simulink model "FOC_ctrl"  (R2025b)
settings: Solver=FixedStepAuto  StartTime=0.0  StopTime=Tstop  FixedStep=p.FastTs  RelTol=1e-3
undefined symbols (not defined in the file): angleDeg, c, Inverter, m, Motor, p, torqueNm, Tstop, we
libraries: simulink x5, fl_lib x4, nesl_utility x3, dspsigops x2, ee_lib x1
(part 2 of 3)

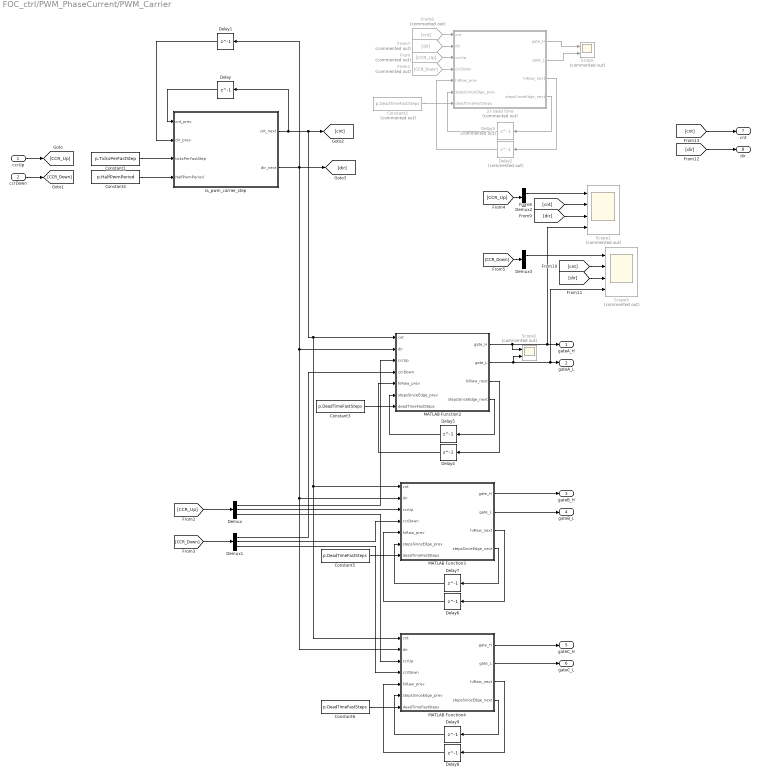
== system FOC_ctrl/PWM_PhaseCurrent/PWM_Carrier ==
  ccrUp : Inport
  ccrDown : Inport  Port=2
  2x dead time : MATLAB Function  Commented=on  TreatAsAtomicUnit=on
  Constant1 : Constant  Value=p.TicksPerFastStep
  Constant2 : Constant  Commented=on  Value=p.DeadTimeFastSteps
  Constant3 : Constant  Value=p.DeadTimeFastSteps
  Constant4 : Constant  Value=p.HalfPwmPeriod
  Constant5 : Constant  Value=p.DeadTimeFastSteps
  Constant6 : Constant  Value=p.DeadTimeFastSteps
  Delay{,4..9} (7 alike) : Delay  DelayLength=1  SampleTime=p.FastTs
  Delay1 : Delay  DelayLength=1  InitialCondition=1  SampleTime=p.FastTs
  Delay2 : Delay  Commented=on  DelayLength=1  SampleTime=p.FastTs
  Delay3 : Delay  Commented=on  DelayLength=1  SampleTime=p.FastTs
  Demux{,1..3} (4 alike) : Demux  Outputs=3
  From : From  Commented=on  GotoTag=CCR_Up
  From1 : From  Commented=on  GotoTag=CCR_Down
  From6 : From  Commented=on  GotoTag=cnt
  From7 : From  Commented=on  GotoTag=dir
  MATLAB Function2 : MATLAB Function  TreatAsAtomicUnit=on
  MATLAB Function3 : MATLAB Function  TreatAsAtomicUnit=on
  MATLAB Function4 : MATLAB Function  TreatAsAtomicUnit=on
  Scope : Scope  Commented=on  NumInputPorts=2
      settings: ActiveDisplayYMinimum=-0.12499999999999997  ActiveDisplayYMaximum=1.125  DataLoggingVariableName=ScopeData14
  Scope1 : Scope  Commented=on  NumInputPorts=4
      settings: ActiveDisplayYMinimum=-9127.6330234277448  ActiveDisplayYMaximum=17916.94761530693  DataLoggingVariableName=ScopeData13
  Scope2 : Scope  Commented=on  NumInputPorts=2
      settings: ActiveDisplayYMinimum=-0.12499999999999997  ActiveDisplayYMaximum=1.125  DataLoggingVariableName=ScopeData21
  Scope5 : Scope  Commented=on  NumInputPorts=4
      settings: ActiveDisplayYMinimum=-665.124999999998  ActiveDisplayYMaximum=5976.1249999999827  DataLoggingVariableName=ScopeData18
  ss_pwm_carrier_step : MATLAB Function  TreatAsAtomicUnit=on
  gateA_H : Outport
  gateA_L : Outport  Port=2
  gateB_H : Outport  Port=3
  gateB_L : Outport  Port=4
  gateC_H : Outport  Port=5
  gateC_L : Outport  Port=6
  cnt : Outport  Port=7
  dir : Outport  Port=8
  wires:
  Constant4/1 -> ss_pwm_carrier_step/4(HalfPwmPeriod)
  Constant1/1 -> ss_pwm_carrier_step/3(ticksPerFastStep)
  Delay/1 -> ss_pwm_carrier_step/1(cnt_prev)
  Delay1/1 -> ss_pwm_carrier_step/2(dir_prev)
  2x dead time/3(hiRaw_next) -> Delay2/1
  Delay2/1 -> 2x dead time/5(hiRaw_prev)
  2x dead time/4(stepsSinceEdge_next) -> Delay3/1
  Delay3/1 -> 2x dead time/6(stepsSinceEdge_prev)
  Constant2/1 -> 2x dead time/7(deadTimeFastSteps)
  2x dead time/1(gate_H) -> Scope/1
  2x dead time/2(gate_L) -> Scope/2
  ccrUp/1 -> [CCR_Up]
  ccrDown/1 -> [CCR_Down]
  From/1 -> 2x dead time/3(ccrUp)
  From1/1 -> 2x dead time/4(ccrDown)
  [CCR_Up] -> Demux/1
  [CCR_Down] -> Demux1/1
  Demux1/1 -> MATLAB Function2/4(ccrDown)
  Demux/1 -> MATLAB Function2/3(ccrUp)
  MATLAB Function2/2(gate_L) -> Scope2/2, Scope5/4, gateA_L/1
  MATLAB Function2/1(gate_H) -> Scope2/1, gateA_H/1, Scope1/4
  Constant3/1 -> MATLAB Function2/7(deadTimeFastSteps)
  Delay5/1 -> MATLAB Function2/6(stepsSinceEdge_prev)
  MATLAB Function2/4(stepsSinceEdge_next) -> Delay5/1
  Delay4/1 -> MATLAB Function2/5(hiRaw_prev)
  MATLAB Function2/3(hiRaw_next) -> Delay4/1
  MATLAB Function3/3(hiRaw_next) -> Delay6/1
  Delay6/1 -> MATLAB Function3/5(hiRaw_prev)
  MATLAB Function3/4(stepsSinceEdge_next) -> Delay7/1
  Delay7/1 -> MATLAB Function3/6(stepsSinceEdge_prev)
  Constant5/1 -> MATLAB Function3/7(deadTimeFastSteps)
  MATLAB Function3/1(gate_H) -> gateB_H/1
  MATLAB Function3/2(gate_L) -> gateB_L/1
  Demux/2 -> MATLAB Function3/3(ccrUp)
  Demux1/2 -> MATLAB Function3/4(ccrDown)
  Demux1/3 -> MATLAB Function4/4(ccrDown)
  Demux/3 -> MATLAB Function4/3(ccrUp)
  MATLAB Function4/2(gate_L) -> gateC_L/1
  MATLAB Function4/1(gate_H) -> gateC_H/1
  Constant6/1 -> MATLAB Function4/7(deadTimeFastSteps)
  Delay9/1 -> MATLAB Function4/6(stepsSinceEdge_prev)
  MATLAB Function4/4(stepsSinceEdge_next) -> Delay9/1
  Delay8/1 -> MATLAB Function4/5(hiRaw_prev)
  MATLAB Function4/3(hiRaw_next) -> Delay8/1
  ss_pwm_carrier_step/2(dir_next) -> [dir], Delay1/1, MATLAB Function2/2(dir), MATLAB Function3/2(dir), MATLAB Function4/2(dir)
  ss_pwm_carrier_step/1(cnt_next) -> MATLAB Function4/1(cnt), MATLAB Function3/1(cnt), MATLAB Function2/1(cnt), [cnt], Delay/1
  [CCR_Up] -> Demux2/1
  [CCR_Down] -> Demux3/1
  Demux2/1 -> Scope1/1
  Demux3/1 -> Scope5/1
  From6/1 -> 2x dead time/1(cnt)
  From7/1 -> 2x dead time/2(dir)
  [cnt] -> Scope1/2
  [dir] -> Scope1/3
  [dir] -> Scope5/3
  [cnt] -> Scope5/2
  [cnt] -> cnt/1
  [dir] -> dir/1

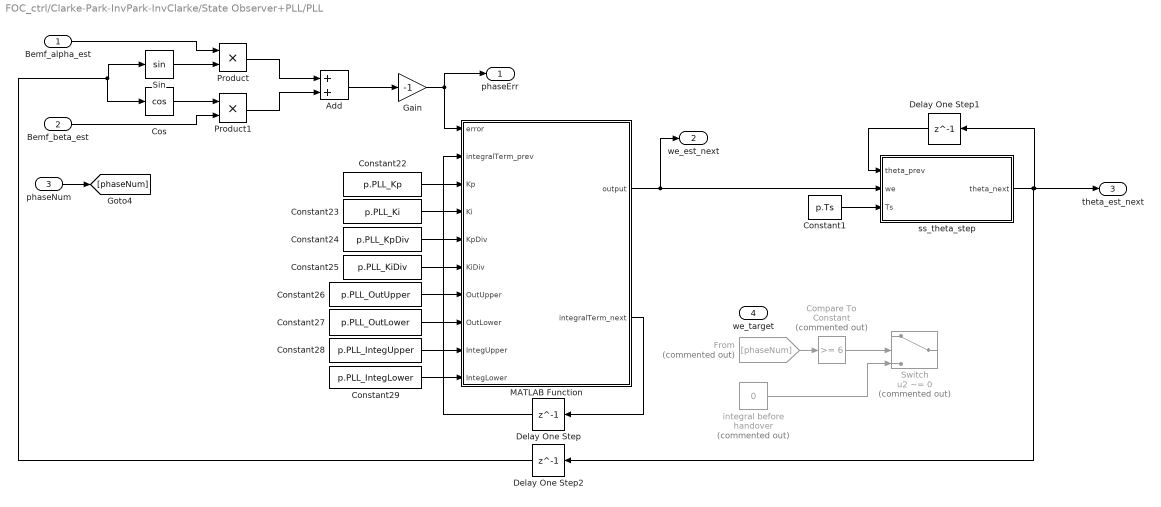
== system FOC_ctrl/Clarke-Park-InvPark-InvClarke/State Observer+PLL/PLL ==
  Bemf_alpha_est : Inport
  Bemf_beta_est : Inport  Port=2
  phaseNum : Inport  Port=3
  we_target : Inport  Port=4
  Add : Sum
  Compare To Constant : simulink/Logic and Bit Operations/Compare To Constant  Commented=on  relop=>=  const=6  OutDataTypeStr=boolean
  Constant1 : Constant  Value=p.Ts
  Constant22 : Constant  Value=p.PLL_Kp
  Constant23 : Constant  Value=p.PLL_Ki
  Constant24 : Constant  Value=p.PLL_KpDiv
  Constant25 : Constant  Value=p.PLL_KiDiv
  Constant26 : Constant  Value=p.PLL_OutUpper
  Constant27 : Constant  Value=p.PLL_OutLower
  Constant28 : Constant  Value=p.PLL_IntegUpper
  Constant29 : Constant  Value=p.PLL_IntegLower
  Cos : Trigonometry  Operator=cos
  Delay One Step : Delay  DelayLength=1
  Delay One Step1 : Delay  DelayLength=1
  Delay One Step2 : Delay  DelayLength=1
  From : From  Commented=on  GotoTag=phaseNum
  Gain : Gain  Gain=-1
  MATLAB Function : MATLAB Function  TreatAsAtomicUnit=on
  Product : Product
  Product1 : Product
  Sin : Trigonometry
  Switch : Switch  Commented=on  Criteria=u2 ~= 0  SaturateOnIntegerOverflow=off  InputSameDT=off
  "integral before handover " : Constant  Commented=on  Value=0
  ss_theta_step : MATLAB Function  TreatAsAtomicUnit=on
  phaseErr : Outport
  we_est_next : Outport  Port=2
  theta_est_next : Outport  Port=3
  wires:
  Add/1 -> Gain/1
  Bemf_beta_est/1 -> Product1/2
  Product1/1 -> Add/2
  Bemf_alpha_est/1 -> Product/1
  Sin/1 -> Product/2
  Product/1 -> Add/1
  Cos/1 -> Product1/1
  Gain/1 -> phaseErr/1, MATLAB Function/1(error)
  Delay One Step2/1 -> Cos/1, Sin/1
  MATLAB Function/2(integralTerm_next) -> Delay One Step/1
  Constant1/1 -> ss_theta_step/3(Ts)
  Delay One Step1/1 -> ss_theta_step/1(theta_prev)
  ss_theta_step/1(theta_next) -> theta_est_next/1, Delay One Step1/1, Delay One Step2/1
  MATLAB Function/1(output) -> we_est_next/1, ss_theta_step/2(we)
  Delay One Step/1 -> MATLAB Function/2(integralTerm_prev)
  Constant29/1 -> MATLAB Function/10(IntegLower)
  Constant28/1 -> MATLAB Function/9(IntegUpper)
  Constant26/1 -> MATLAB Function/7(OutUpper)
  Constant27/1 -> MATLAB Function/8(OutLower)
  Constant25/1 -> MATLAB Function/6(KiDiv)
  Constant24/1 -> MATLAB Function/5(KpDiv)
  Constant23/1 -> MATLAB Function/4(Ki)
  Constant22/1 -> MATLAB Function/3(Kp)
  From/1 -> Compare To Constant/1
  "integral before handover "/1 -> Switch/3
  Compare To Constant/1 -> Switch/2
  phaseNum/1 -> [phaseNum]

== system FOC_ctrl/Cogging Torque/Variant Subsystem/BD Nano ==
  theta : Inport
  BD Nano : MATLAB Function  TreatAsAtomicUnit=on  VariantControl=Option.Product==1
  Gain : Gain  Gain=c.ENABLE_COGGING_TORQUE
  Tcog : Outport
  wires:
  BD Nano/1(Tcog) -> Gain/1
  theta/1 -> BD Nano/1(theta)
  Gain/1 -> Tcog/1

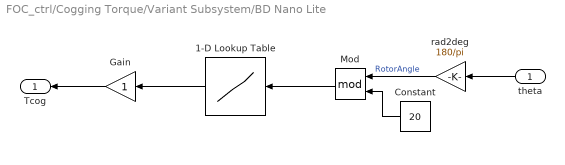
== system FOC_ctrl/Cogging Torque/Variant Subsystem/BD Nano Lite ==
  theta : Inport
  1-D Lookup Table : Lookup_n-D  NumberOfTableDimensions=1  BreakpointsForDimension1=|  BreakpointsForDimension1FirstPoint=0  BreakpointsForDimension1Spacing=0.5  Table=|  InterpMethod=Cubic spline  ExtrapMethod=Cubic spline  InternalRulePriority=Speed  RndMeth=Simplest
      BreakpointsForDimension1=|
      | [0.0
      | 0.5
      | 1.0
      | 1.5
      | 2.0
      | 2.5
      | 3.0
      | 3.5
      | 4.0
      | 4.5
      | 5.0
      | 5.5
      | 6.0
      | 6.5
      | 7.0
      | 7.5
      | 8.0
      | 8.5
      | 9.0
      | 9.5
      | 10.0
      | 10.5
      | 11.0
      | 11.5
      | 12.0
      | 12.5
      | 13.0
      | 13.5
      | 14.0
      | 14.5
      | 15.0
      | 15.5
      | 16.0
      | 16.5
      | 17.0
      | 17.5
      | 18.0
      | 18.5
      | 19.0
      | 19.5
      | 20.0]
      Table=|
      | [0.001
      | 0.002
      | 0.003
      | 0.004
      | 0.005
      | 0.007
      | 0.009
      | 0.011
      | 0.013
      | 0.015
      | 0.017
      | 0.018
      | 0.019
      | 0.018
      | 0.016
      | 0.013
      | 0.010
      | 0.007
      | 0.005
      | 0.003
      | 0.002
      | 0.001
      | 0.000
      | -0.002
      | -0.004
      | -0.007
      | -0.010
      | -0.014
      | -0.017
      | -0.019
      | -0.020
      | -0.019
      | -0.018
      | -0.016
      | -0.014
      | -0.012
      | -0.010
      | -0.008
      | -0.006
      | -0.004
      | -0.001]
  Constant : Constant  Value=20
  Gain : Gain
  Mod : Math  Operator=mod
  rad2deg : Gain  Gain=180/pi
  Tcog : Outport
  wires:
  theta/1 -> rad2deg/1
  1-D Lookup Table/1 -> Gain/1
  Mod/1 -> 1-D Lookup Table/1
  rad2deg/1 -> Mod/1  "RotorAngle"
  Constant/1 -> Mod/2
  Gain/1 -> Tcog/1

== matlab function FOC_ctrl/PWM_PhaseCurrent/get_phase_currents ==
  data: sector input; ia output; iflag input; JDR1 input; JDR2 input; alignFlag input; offset input; convFactorInv input; IaEst input; IbEst input; IcEst input; ib output; ic output
function [ia, ib, ic] = ss_get_phase_currents(sector, iflag, JDR1, JDR2, alignFlag, ...
    offset, convFactorInv, IaEst, IbEst, IcEst)
%SS_GET_PHASE_CURRENTS MATLAB port of R1_GetPhaseCurrents()
% (Src/r1_ps_pwm_curr_fdbk.c, ~lines 463-866).
%
% Reconstructs ia, ib (ic follows from KCL, ia+ib+ic=0) from the two raw
% ADC codes taken this PWM period, using:
%   - sector           : which of the six switching patterns is active
%   - iflag            : IA_OK/IB_OK/IC_OK bits from
%                        ss_calc_duty_and_samplepoints - which of the two
%                        phase currents this sector could sample were
%                        actually inside a wide-enough (>=TMin) window
%   - alignFlag        : true only during the fixed-angle rotor alignment
%                        step at startup (angle pinned to a sector
%                        midpoint, e.g. 30 deg for sector 1) - in that
%                        special case the un-sampled phase's current is
%                        known to be exactly 0 instead of needing an
%                        estimate
%   - IaEst/IbEst/IcEst: fallback current estimates (in the firmware these
%                        come from pwm_curr_fdbk.c's Clarke-transform of
%                        the FOC's own alpha-beta current reference, i.e.
%                        "the current we commanded", used whenever this
%                        period's real sample(s) aren't trustworthy)
%
% Three outcomes per sector, exactly mirroring the C switch/if structure:
%   1) BOTH of the sector's two candidate phases are flagged OK
%        -> both come from real ADC samples this period (best case)
%   2) ONE of the two is flagged OK
%        -> that one is a real sample; the other phase is either forced
%           to 0 (during alignment) or taken from the estimate
%   3) NEITHER is flagged OK
%        -> both phases fall back to the estimate entirely (no real
%           sample was usable this period at all)
%
% JDR1/JDR2 are raw ADC codes (offset not yet removed); convFactorInv is
% CURRENT_CONV_FACTOR_INV (Amps per ADC digit). This port converts to Amps
% immediately after offset removal (wAux1/wAux2), so the branch algebra
% below is unit-for-unit identical to the C source, just already in Amps
% instead of raw int16 digits.

IA_OK = uint8(1); IB_OK = uint8(2); IC_OK = uint8(4);

wAux1 = (double(JDR1) - offset) * convFactorInv;
wAux2 = (double(JDR2) - offset) * convFactorInv;

ia = 0; ib = 0; ic = 0;

switch sector
    case 1
        pair = bitand(iflag, bitor(IA_OK, IC_OK));
        if pair == bitor(IA_OK, IC_OK)
            ia = wAux2; ic = -wAux1; ib = -ia - ic;
        elseif pair ~= 0
            if alignFlag                                   % START Position, 30 deg
                if pair == IA_OK, ia = wAux2; ib = 0; ic = -ia;
                else,             ic = -wAux1; ia = -ic; ib = 0;
                end
            else
                if pair == IA_OK, ia = wAux2; ib = IbEst; ic = -ia - ib;
                else,             ic = -wAux1; ib = IbEst; ia = -ib - ic;
                end
            end
        else
            ia = IaEst; ic = IcEst; ib = -ia - ic;
        end

    case 2
        pair = bitand(iflag, bitor(IB_OK, IC_OK));
        if pair == bitor(IB_OK, IC_OK)
            ib = wAux2; ic = -wAux1; ia = -ib - ic;
        elseif pair ~= 0
            if alignFlag                                   % START Position, 90 deg
                if pair == IB_OK, ib = wAux2; ia = 0; ic = -ib;
                else,             ic = -wAux1; ia = 0; ib = -ic;
                end
            else
                if pair == IB_OK, ib = wAux2; ia = IaEst; ic = -ia - ib;
                else,             ic = -wAux1; ia = IaEst; ib = -ia - ic;
                end
            end
        else
            ib = IbEst; ic = IcEst; ia = -ib - ic;
        end

    case 3
        pair = bitand(iflag, bitor(IA_OK, IB_OK));
        if pair == bitor(IA_OK, IB_OK)
            ib = wAux2; ia = -wAux1;
        elseif pair ~= 0
            if alignFlag                                   % START Position, 150 deg
                if pair == IB_OK, ib = wAux2; ia = -ib;
                else,             ia = -wAux1; ib = -ia;
                end
            else
                if pair == IB_OK, ib = wAux2; ia = IaEst;
                else,             ia = -wAux1; ib = IbEst;
                end
            end
        else
            ib = IbEst; ia = IaEst;
        end
        ic = -ia - ib;  % not computed by the C fn here (ab_t has no `c`); KCL added for convenience

    case 4
        pair = bitand(iflag, bitor(IA_OK, IC_OK));
        if pair == bitor(IA_OK, IC_OK)
            ia = -wAux1; ic = wAux2; ib = -ia - ic;
        elseif pair ~= 0
            if alignFlag                                   % START Position, 210 deg
                if pair == IC_OK, ic = wAux2; ia = -ic; ib = 0;
                else,             ia = -wAux1; ib = 0;
                end
            else
                if pair == IC_OK, ic = wAux2; ib = IbEst; ia = -ib - ic;
                else,             ia = -wAux1; ib = IbEst;
                end
            end
        else
            ic = IcEst; ia = IaEst; ib = -ia - ic;
        end

    case 5
        pair = bitand(iflag, bitor(IB_OK, IC_OK));
        if pair == bitor(IB_OK, IC_OK)
            ib = -wAux1; ic = wAux2; ia = -ib - ic;
        elseif pair ~= 0
            if alignFlag                                   % START Position, 270 deg
                if pair == IC_OK, ic = wAux2; ia = 0; ib = -ic;
                else,             ib = -wAux1; ia = 0;
                end
            else
                if pair == IC_OK, ic = wAux2; ia = IaEst; ib = -ia - ic;
                else,             ib = -wAux1; ia = IaEst;
                end
            end
        else
            ic = IcEst; ib = IbEst; ia = -ib - ic;
        end

    case 6
        pair = bitand(iflag, bitor(IA_OK, IB_OK));
        if pair == bitor(IA_OK, IB_OK)
            ia = wAux2; ib = -wAux1;
        elseif pair ~= 0
            if alignFlag                                   % START Position, 330 deg
                if pair == IA_OK, ia = wAux2; ib = -ia;
                else,             ib = -wAux1; ia = -ib;
                end
            else
                if pair == IA_OK, ia = wAux2; ib = IbEst;
                else,             ib = -wAux1; ia = IaEst;
                end
            end
        else
            ia = IaEst; ib = IbEst;
        end
        ic = -ia - ib;  % not computed by the C fn here (ab_t has no `c`); KCL added for convenience

    otherwise
        error('ss_get_phase_currents:sector', 'sector must be 1..6');
end

end

== matlab function FOC_ctrl/Cogging Torque/Variant Subsystem/BD Nano/BD Nano ==
  data: theta input size=1; Tcog output size=1
function Tcog = fcn(theta)

Tcog = 0.039*sin(18*theta);

== matlab function FOC_ctrl/PWM_PhaseCurrent/ADC_trigger ==
  data: cnt input; trig1 output; dir input; SamplePoint1 input; SamplePoint2 input; ticksPerFastStep input; trig2 output
function [trig1, trig2] = ss_adc_trigger_step(cnt, dir, SamplePoint1, SamplePoint2, ticksPerFastStep)
%SS_ADC_TRIGGER_STEP One fast-rate (p.FastTs) step of the TIM1 CH5/CH6 ->
% TRGO2 -> ADC-injected-trigger chain. Replaces the "SamplePoint changed"
% detector, which fired both triggers simultaneously at the period boundary.
%
% ---------------------------------------------------------------------------
% What the hardware actually does (verified against this build's firmware)
% ---------------------------------------------------------------------------
% Src/main.c, MX_TIM1_Init():
%   CounterMode        = TIM_COUNTERMODE_CENTERALIGNED2
%   CH5, CH6 OCMode    = TIM_OCMODE_PWM2      <-- note: PWM mode *2*
%   MasterOutputTrigger2 = TIM_TRGO2_OC5REF_RISING_OC6REF_RISING
% Src/main.c, ADC2 injected config:
%   ExternalTrigInjecConv = ADC_EXTERNALTRIGINJEC_T1_TRGO, 2 conversions
% Src/r1_ps_pwm_curr_fdbk.c, R1_CalcDutyCycles() (~line 1259):
%   CCR5 = SamplePoint1,  CCR6 = SamplePoint2
%
% In PWM mode 2 the reference OCxREF is LOW while CNT < CCRx and HIGH while
% CNT > CCRx. So an OCxREF *rising* edge is an UP-COUNT crossing of CCRx.
% Both conversions therefore happen in the UP-COUNTING half of the
% center-aligned period, SamplePoint1 first (it is the lower value), then
% SamplePoint2 -> injected rank 1 = JDR1 = SamplePoint1, rank 2 = JDR2 =
% SamplePoint2. That is exactly the pairing ss_get_phase_currents assumes
% (JDR1 -> low-duty phase, JDR2 -> high-duty phase).
%
% This also explains the asymmetric shift: aShiftval is applied +shift in the
% up half (DmaBuffCCR[0:2]) and -shift in the down half (DmaBuffCCR[4:6]), and
% is only ever applied to the max- or min-duty phase, never the mid one. The up
% half is where the shift WIDENS both sampling windows; the down half pays it
% back so the average duty (= commanded voltage) is unchanged. Nothing is
% sampled in the down half, so the narrowed windows there do not matter.
%
% ---------------------------------------------------------------------------
% Why the sample point must be snapped DOWN to the fast grid
% ---------------------------------------------------------------------------
% The simulated carrier only takes values that are multiples of
% ticksPerFastStep (= p.TicksPerFastStep, 170 ticks = 1 us at the current
% settings), so the gate edges - and therefore the real sampling windows in
% the simulation - are quantized to that grid too.
%
% SamplePoint1 = CCR_mid - TSample sits only TSample = 41 ticks (0.24 fast
% steps) below the mid-phase edge. If you fire on the FIRST grid point at or
% after SamplePoint1, that grid point coincides with the mid-phase edge
% whenever (CCR_mid mod ticksPerFastStep) > TSample - i.e. 76% of the time -
% and you sample the wrong window, inside the dead time.
%
% Firing on the LAST grid point at or before the sample point instead is
% provably inside the correct window for every duty pattern the firmware
% flags as valid (windows are guaranteed >= TMin = 415 ticks wide, and
% snapping down costs at most ticksPerFastStep-1 = 169 ticks). Run
% ss_adc_timing_report to re-verify this after any change to PWM_FREQUENCY,
% p.PwmCarrierSamplesPerPeriod or p.DeadTime_ns.
%
% ---------------------------------------------------------------------------
% Inputs / outputs
% ---------------------------------------------------------------------------
% cnt, dir          : ss_pwm_carrier_step.m outputs, THIS fast step
% SamplePoint1/2    : ss_calc_duty_and_samplepoints.m outputs, in timer ticks,
%                     held constant over the PWM period (p.Ts rate signal,
%                     zero-order-held into this fast-rate subsystem)
% ticksPerFastStep  : p.TicksPerFastStep
%
% trig1, trig2      : one-fast-step pulses for the two Sample and Hold
%                     blocks (JDR1 <- trig1, JDR2 <- trig2). No state is
%                     needed: each sample point is bracketed by exactly one
%                     up-count step, so each pulse fires exactly once per
%                     PWM period.
%
% NOTE: the gate vector reaches the Simscape inverter one fast step late
% (Delay6elements at the model root), so Vamp_out at step k reflects the
% carrier value at step k-1. Delay trig1/trig2 by p.AdcTrigAlignSteps fast
% steps OUTSIDE this function to line them up - see the header of
% ss_adc_timing_report for how to check the alignment on a scope.

upCounting = dir > 0;

trig1 = upCounting && (cnt <= SamplePoint1) && ((cnt + ticksPerFastStep) > SamplePoint1);
trig2 = upCounting && (cnt <= SamplePoint2) && ((cnt + ticksPerFastStep) > SamplePoint2);

end

== matlab function FOC_ctrl/Clarke-Park-InvPark-InvClarke/Park ==
  data: Ialpha input; Id output; Ibeta input; theta input; Iq output
function [Id, Iq] = ss_park(Ialpha, Ibeta, theta)
%SS_PARK MATLAB port of MCM_Park() (Src/mc_math.c, ~lines 143-239).
%
% Same sin/cos role-swap as the firmware (Iq uses cos, Id uses sin) -
% verified as the exact inverse of ss_rev_park.m under this convention
% (see ss_clarke.m header). theta is the rotor electrical angle in
% radians (the firmware's Theta is the same angle in Q1.15 format via a
% trig LUT - using cos/sin directly here is the floating-point
% equivalent).
%
% Ialpha, Ibeta : stationary frame currents (ss_clarke.m output)
% theta         : rotor electrical angle, radians
% Id, Iq        : synchronous (rotor) frame currents

c = cos(theta);
s = sin(theta);

Iq = Ialpha * c - Ibeta * s;
Id = Ialpha * s + Ibeta * c;

end

== matlab function FOC_ctrl/Clarke-Park-InvPark-InvClarke/Clarke ==
  data: Ia input; Ialpha output; Ib input; Ibeta output
function [Ialpha, Ibeta] = ss_clarke(Ia, Ib)
%SS_CLARKE MATLAB port of MCM_Clarke() (Src/mc_math.c, ~lines 71-100).
%
% Note this firmware's beta axis is flipped in sign relative to the
% "textbook" amplitude-invariant Clarke transform (which would be
% Ibeta = +(Ia+2*Ib)/sqrt(3)) - this is a deliberate, consistent ST
% convention: MCM_Park/MCM_Rev_Park are written to be exact inverses of
% each other under THIS sign (verified algebraically), so as long as
% ss_park.m / ss_rev_park.m match it too, the closed loop is self-
% consistent - only the direction label ("beta") differs from other
% textbooks, not the actual closed-loop behavior.
%
% Ia, Ib : measured phase currents (from the single-shunt reconstruction,
%          i.e. this model's Ia/Ib outputs)
% Ialpha, Ibeta : stationary (alpha-beta) frame currents

Ialpha = Ia;
Ibeta  = -(Ia + 2*Ib) / sqrt(3);

end

== matlab function FOC_ctrl/Clarke-Park-InvPark-InvClarke/rev_park ==
  data: Vd input; Valpha output; Vq input; theta input; Vbeta output
function [Valpha, Vbeta] = ss_rev_park(Vd, Vq, theta)
%SS_REV_PARK MATLAB port of MCM_Rev_Park() (Src/mc_math.c, ~lines
% 258-297): Valpha = Vq*cos(theta) + Vd*sin(theta)
%           Vbeta  = -Vq*sin(theta) + Vd*cos(theta)
%
% Exact inverse of ss_park.m under the same convention (verified when
% Park was written: Rev_Park(Park(Ialpha,Ibeta,theta),theta) = Ialpha,
% Ibeta for any theta).
%
% Vd, Vq : synchronous-frame voltage commands (PI controller outputs,
%          already converted to per-unit via p.VoltageFullScale)
% theta  : rotor electrical angle, radians (same theta fed to ss_park.m)

c = cos(theta);
s = sin(theta);

Valpha = Vq * c + Vd * s;
Vbeta  = -Vq * s + Vd * c;

end

== matlab function FOC_ctrl/Clarke-Park-InvPark-InvClarke/inv_clarke(V) ==
  data: Valpha input; Va output; Vbeta input; Vb output; Vc output
function [Va, Vb, Vc] = ss_inv_clarke(Valpha, Vbeta)
%SS_INV_CLARKE Inverse Clarke transform - NOT a firmware port (the real
% MCSDK has no such function: PWMC_SetPhaseVoltage() computes SVM duty
% directly from alpha-beta via the fixed-point wX/wY/wZ method, never
% forming Va/Vb/Vc explicitly). This is the bridge WE need because
% ss_svpwm_minmax.m (the SVPWM stage already validated in this build)
% works in the three-phase domain rather than being a byte-for-byte port
% of that alpha-beta-native method (see ss_sector_from_duty.m header).
%
% Derived as the exact algebraic inverse of ss_clarke.m's specific sign
% convention (Ibeta = -(Ia+2*Ib)/sqrt(3), i.e. flipped vs. the "textbook"
% Clarke transform) - NOT copied from a generic inverse-Clarke formula,
% to guarantee round-tripping through ss_clarke.m -> ss_park.m ->
% ss_rev_park.m -> here reproduces the original three phases exactly.
% Verified: ss_inv_clarke(ss_clarke(Ia,Ib)) == [Ia, Ib, Ic] for any Ia,Ib.
%
% Valpha, Vbeta : ss_rev_park.m output (per-unit stationary-frame voltage)
% Va, Vb, Vc    : per-unit three-phase reference voltage, same scale/sign
%                 convention as the Va/Vb/Vc already feeding
%                 ss_svpwm_minmax.m

Va = Valpha;
Vb = -Valpha/2 - (sqrt(3)/2) * Vbeta;
Vc = -Valpha/2 + (sqrt(3)/2) * Vbeta;

end

== matlab function FOC_ctrl/Clarke-Park-InvPark-InvClarke/Startup/the phase sequencer_Updated ==
  data: t_elapsed input; we_target output; Idref_phase output; Iqref_phase output; phaseNum output; p parameter
function [we_target, Idref_phase, Iqref_phase, phaseNum] = ss_startup_sequencer(t_elapsed, p)
%SS_STARTUP_SEQUENCER Smooth-transition startup sequencer for loaded motor
%
% Phase Breakdown:
%   Phase 1 (Align)       : 0.000 - 0.200 s | Holds 0 RPM | Id = 10A, Iq = 0A
%   Phase 1.5 (Transition): 0.200 - 0.220 s | Holds 0 RPM | Id ramps 10A->0A, Iq ramps 0A->10A
%   Phase 2 (Ramp/Acc)    : 0.220 - 0.620 s | Ramps to 2500 RPM | Iq tapers 10A->8A
%   Phase 3               : 0.620 - 0.621 s | Ramps to 2510 RPM | Iq = 8A
%   Phase 4               : 0.621 - 0.622 s | Ramps to 2520 RPM | Iq = 8A
%   Phase 5               : 0.622 - 0.623 s | Ramps to 2530 RPM | Iq = 8A
%   Phase 6               : > 0.623 s       | Ready for closed-loop handover

rpm2we = (2*pi/60) * p.MotorPolePairs;
we_bkpts = p.Startup_RPM * rpm2we;
t_bkpts  = [0, p.Startup_T];

% 1. Command open-loop target electrical speed (we_target)
t_clamped = min(t_elapsed, p.Startup_T(end));
we_target = interp1(t_bkpts, we_bkpts, t_clamped, 'linear');

% 2. Current Reference and Phase State Machine
T_align = p.Startup_T(1); % End of pure align
T_blend = p.Startup_T(2); % End of Id -> Iq blend duration

if t_elapsed <= T_align
    % --- PHASE 1: Pure Alignment (DC Lock) ---
    phaseNum = 1;
    Idref_phase = p.Startup_Id_A;
    Iqref_phase = 0;

elseif t_elapsed <= T_blend
    % --- PHASE 1.5: Smooth Vector Blend (Soft-Transfer at Standstill) ---
    phaseNum = 1.5;
    % Normalized alpha factor going from 0 -> 1 over the blend time
    alpha = (t_elapsed - T_align) / (T_blend - T_align);
    
    % Smooth cross-fade between Id and Iq to avoid current step spikes
    Idref_phase = (1 - alpha) * p.Startup_Id_A;
    Iqref_phase = alpha * p.Startup_Iq_Breakaway_A;

elseif t_elapsed <= p.Startup_T(3)
    % --- PHASE 2: Main Acceleration Ramp ---
    phaseNum = 2;
    Idref_phase = 0;
    
    % Taper Iq down from Breakaway Torque (10A) to Running Startup Torque (4A)
    % as speed increases and static friction drops to dynamic friction
    T_ramp_start = T_blend;
    T_ramp_end   = p.Startup_T(3);
    beta = (t_elapsed - T_ramp_start) / (T_ramp_end - T_ramp_start);
    
    Iqref_phase = (1 - beta) * p.Startup_Iq_Breakaway_A + beta * p.Startup_Iq_A;

elseif t_elapsed <= p.Startup_T(4)
    % --- PHASE 3 ---
    phaseNum = 3;
    Idref_phase = 0;
    Iqref_phase = p.Startup_Iq_A;

elseif t_elapsed <= p.Startup_T(5)
    % --- PHASE 4 ---
    phaseNum = 4;
    Idref_phase = 0;
    Iqref_phase = p.Startup_Iq_A;

elseif t_elapsed <= p.Startup_T(6)
    % --- PHASE 5 ---
    phaseNum = 5;
    Idref_phase = 0;
    Iqref_phase = p.Startup_Iq_A;

else
    % --- PHASE 6: Observer Handoff Ready ---
    phaseNum = 6;
    Idref_phase = 0;
    Iqref_phase = p.Startup_Iq_A; % Holds constant; superseded by Speed Loop Iqref once closed
end

end

== matlab function FOC_ctrl/Clarke-Park-InvPark-InvClarke/State Observer+PLL/MATLAB Function ==
  data: we_est input; speedErrPct output; we_target input; tolFrac input; isConverged output
function [speedErrPct, isConverged] = check_convergence(we_est, we_target, tolFrac)
% tolFrac: e.g. 0.05 for 5%
if abs(we_target) > 50   % avoid a meaningless % error near standstill
    speedErrPct = abs(we_est - we_target) / abs(we_target) * 100;
else
    speedErrPct = 999;    % force "not converged" at/near standstill
end
isConverged = speedErrPct < (tolFrac*100);
end

== matlab function FOC_ctrl/Clarke-Park-InvPark-InvClarke/CalcPhaseCurrentsEst ==
  data: Iq input; IaEst output; Id input; IqAvg_prev input; IdAvg_prev input; theta input; IbEst output; IcEst output; IqAvg_next output; IdAvg_next output; p parameter
function [IaEst, IbEst, IcEst, IqAvg_next, IdAvg_next] = ...
    ss_calc_phase_currents_est(Iq, Id, IqAvg_prev, IdAvg_prev, theta, p)
%SS_CALC_PHASE_CURRENTS_EST MATLAB port of PWMC_CalcPhaseCurrentsEst()
% (Src/pwm_curr_fdbk.c, ~lines 489-529), called once per PWM period from
% Src/mc_tasks_foc.c:787 - the real firmware's replacement for a naive
% sample-and-hold fallback estimate.
%
% NOT built from the current reference (a simplification I mistakenly
% described earlier) - it's built from the MEASURED Iq/Id (this period's
% ss_park output, i.e. the just-reconstructed current), lightly low-pass
% filtered, then rotated back through Rev_Park + inverse-Clarke into an
% a/b/c estimate. This gives a smoother, more physically continuous
% fallback than repeating a single stale sample, without needing to know
% anything about what the controller commanded.
%
% PWMC_LowPassFilter()'s Q15 fixed-point accumulator recursion simplifies
% (once you divide through by the 32768 scaling) to the standard
% exponential filter used here: Y[k] = Y[k-1] + alpha*(in[k]-Y[k-1]),
% alpha = p.LPFAlpha (~0.5 - LPF_FILT_CONST/32768 - a light filter, not
% heavy smoothing).
%
% ss_rev_park.m and ss_inv_clarke.m are reused as-is: Rev_Park is just a
% rotation (works on filtered Id/Iq exactly like it works on PI voltage
% output), and the firmware's temp1/temp2 "Reverse Clarke" formula here
% is, term for term, identical to ss_inv_clarke.m (already verified when
% that file was written).
%
% TIMING: in the C code, PWMC_GetPhaseCurrents() (which reads
% pHandle->IaEst) runs BEFORE PWMC_CalcPhaseCurrentsEst() (which writes
% it) within the same period - so GetPhaseCurrents always sees LAST
% period's estimate, never this period's freshly computed one. Replicate
% this by feeding IaEst/IbEst/IcEst back into ss_get_phase_currents.m
% through a Unit Delay (Z^-1), NOT directly - otherwise this creates the
% same zero-delay algebraic loop we already had to fix once for the
% Vd/Vq path.
%
% Iq, Id             : measured synchronous-frame current (ss_park output,
%                      THIS period)
% IqAvg_prev/IdAvg_prev : filter state - feed back through two Unit Delay
%                      (Z^-1) blocks, initial condition 0
% theta              : rotor electrical angle, radians (same theta used
%                      elsewhere - the real firmware uses hElAngle with an
%                      extra speed-compensation term here that this
%                      simplified open-loop-theta build doesn't model)
%
% IaEst,IbEst,IcEst  : feed through THREE MORE Unit Delay (Z^-1) blocks
%                      before wiring into ss_get_phase_currents.m's
%                      IaEst/IbEst/IcEst inputs (see TIMING note above)
% IqAvg_next/IdAvg_next : feed back to IqAvg_prev/IdAvg_prev next period

IqAvg_next = IqAvg_prev + p.LPFAlpha * (Iq - IqAvg_prev);
IdAvg_next = IdAvg_prev + p.LPFAlpha * (Id - IdAvg_prev);

[Ialpha_est, Ibeta_est] = ss_rev_park(IdAvg_next, IqAvg_next, theta);
[IaEst, IbEst, IcEst] = ss_inv_clarke(Ialpha_est, Ibeta_est);

end

== matlab function FOC_ctrl/Clarke-Park-InvPark-InvClarke/State Observer+PLL/PLL/MATLAB Function ==
  data: error input; integralTerm_prev input; Kp input; Ki input; KpDiv input; KiDiv input; OutUpper input; OutLower input; IntegUpper input; IntegLower input; output output; integralTerm_next output
function [output, integralTerm_next] = ss_pi_controller(error, integralTerm_prev, ...
    Kp, Ki, KpDiv, KiDiv, OutUpper, OutLower, IntegUpper, IntegLower)
%SS_PI_CONTROLLER MATLAB port of PI_Controller()
% (MCSDK_v6.4.2-Full/MotorControl/MCSDK/MCLib/Any/Src/pid_regulator.c,
% ~lines 622-738). Used for both the Id and Iq current loops (same
% function, different gains - matches how the firmware reuses one
% PI_Controller() for pPIDId[M1] and pPIDIq[M1]).
%
% Structure: proportional term, integral term (accumulated then clamped
% to [IntegLower,IntegUpper] BEFORE being added to the proportional
% term), summed and clamped to [OutLower,OutUpper] - then, distinctively,
% whatever amount was clamped off ("discharge") is fed back and added to
% the stored integral term. That's back-calculation anti-windup: it stops
% the integrator winding up further while the output is saturated,
% without needing a separate windup-detection flag.
%
% NOT ported: the C code's wIntegral_sum_temp int32-overflow guards
% (lines ~654-689) - those exist to protect a 32-bit fixed-point
% accumulator from wrapping around, which isn't a concern in double-
% precision floating point. The control algorithm itself (this function)
% is unaffected by omitting them.
%
% integralTerm_prev/integralTerm_next : the PI's stored integral state
% (pHandle->wIntegralTerm) - feed back through a Unit Delay (Z^-1),
% initial condition 0, same pattern as IaEst/IbEst/IcEst and theta_prev
% elsewhere in this build.
%
% error : reference - measured, in the SAME units the gains were tuned
%         for - i.e. raw ADC-digit-equivalent current, NOT Amps (see
%         ss_params.m's "Current-loop PI gains" section for the Amps<->
%         digit and per-unit-voltage<->raw conversions to do at the call
%         site).
% Kp, Ki, KpDiv, KiDiv, OutUpper, OutLower, IntegUpper, IntegLower :
%         p.IQ_* / p.ID_* / p.PI_* from ss_params.m

propTerm = Kp * error;

if Ki == 0
    integralTerm = 0;
else
    integralSum = integralTerm_prev + Ki * error;
    if integralSum > IntegUpper
        integralTerm = IntegUpper;
    elseif integralSum < IntegLower
        integralTerm = IntegLower;
    else
        integralTerm = integralSum;
    end
end

output_raw = propTerm / KpDiv + integralTerm / KiDiv;

discharge = 0;
if output_raw > OutUpper
    discharge = OutUpper - output_raw;
    output = OutUpper;
elseif output_raw < OutLower
    discharge = OutLower - output_raw;
    output = OutLower;
else
    output = output_raw;
end

integralTerm_next = integralTerm + discharge * KiDiv;

end

== matlab function FOC_ctrl/Clarke-Park-InvPark-InvClarke/Startup/handover_timing_gate ==
  data: we_est input; T5_eff output; we_target input; t_elapsed input; tolFrac input; minRampTime input; timeoutMargin input; T5_fixed input; minSpeed input; Count output
function [T5_eff, Count]= handover_timing_gate(we_est, we_target, t_elapsed, tolFrac, minRampTime, timeoutMargin, T5_fixed, minSpeed)
persistent okCount tLatched
if isempty(okCount)
    okCount  = 0;
    tLatched = -1;
end

DEBOUNCE_N = 20;  % consecutive in-tolerance samples required (~1.6ms @ 12.5kHz)

if t_elapsed >= minRampTime && abs(we_target) > 50 && abs(we_est) > minSpeed
    speedErrPct = abs(we_est - we_target) / abs(we_target) * 100;
    if speedErrPct < tolFrac*100
        okCount = okCount + 1;
    else
        okCount = 0;
    end
else
    okCount = 0;
end
Count=okCount;
if tLatched < 0 && okCount >= DEBOUNCE_N
    tLatched = t_elapsed;          % latch the instant convergence was confirmed
end

if tLatched < 0 && okCount >= DEBOUNCE_N
    tLatched = t_elapsed;                   % genuine convergence, latched
elseif tLatched < 0 && t_elapsed >= (T5_fixed + timeoutMargin)
    tLatched = T5_fixed + timeoutMargin;    % timeout fallback, latched to a FIXED point
end

if tLatched >= 0
    T5_eff = tLatched;
else
    T5_eff = 1e6;
end

end

== matlab function FOC_ctrl/Clarke-Park-InvPark-InvClarke/modulation_index(Investigation only) ==
  data: Va input; m output; Vb input; Vc input
function m = ss_modulation_index(Va, Vb, Vc)
%SS_MODULATION_INDEX Voltage vector magnitude (the effective modulation
% index "m") recovered from the three per-unit phase voltages feeding
% ss_svpwm_minmax.m - a diagnostic, not a firmware port.
%
% Derived as the algebraic inverse of ss_inv_clarke.m's specific
% convention (Va=Valpha, Vb=-Valpha/2-sqrt(3)/2*Vbeta,
% Vc=-Valpha/2+sqrt(3)/2*Vbeta => Vbeta=(Vc-Vb)/sqrt(3)), NOT a generic
% formula, so it stays consistent with this build's sign convention.
%
% Simpler equivalent (no need to wait until after InvClarke): since
% ss_rev_park.m is a pure rotation, it preserves vector magnitude, so
% m = sqrt(Vd^2+Vq^2) computed directly from the (per-unit) PI outputs
% gives the exact same number - check there instead if it's more
% convenient to scope.
%
% Guide values: m <= 1.0 is the plain sine-triangle linear range;
% 1.0 < m <= 2/sqrt(3) ~= 1.1547 is the extended range the min-max
% injection in ss_svpwm_minmax.m buys you (six-step limit); m above that
% means the commanded voltage vector can no longer be tracked - the
% actual output will be less than/distorted relative to what was
% commanded (overmodulation).

Valpha = Va;
Vbeta = (Vc - Vb) / sqrt(3);

m = sqrt(Valpha.^2 + Vbeta.^2);

end

== matlab function FOC_ctrl/PWM_PhaseCurrent/PWM_Carrier/ss_pwm_carrier_step ==
  data: cnt_prev input; cnt_next output; dir_prev input; ticksPerFastStep input; HalfPwmPeriod input; dir_next output
function [cnt_next, dir_next] = ss_pwm_carrier_step(cnt_prev, dir_prev, ticksPerFastStep, HalfPwmPeriod)
%SS_PWM_CARRIER_STEP One fast-rate (p.FastTs) step of the real TIM1
% center-aligned up-down counter, running underneath the whole p.Ts-rate
% model - NOT a firmware port (the real counter is free-running hardware,
% not software), just this simulation's stand-in for it.
%
% Advances the counter by ticksPerFastStep each fast step and reflects
% direction at 0 and HalfPwmPeriod, producing the same triangle-wave
% counter TIM1 actually runs (0 -> HalfPwmPeriod -> 0, repeating every
% p.Ts). Run this in a subsystem at p.FastTs (see ss_params.m's "PWM
% carrier" section) - NOT at the model's main p.Ts rate.
%
% cnt_prev, dir_prev : counter state (ticks, +1/-1) - feed back through
%                       two Unit Delay (Z^-1) blocks AT THE FAST RATE,
%                       initial condition cnt=0, dir=+1
% ticksPerFastStep    : p.TicksPerFastStep
% HalfPwmPeriod       : p.HalfPwmPeriod (ARR, timer ticks)

cnt_raw = cnt_prev + dir_prev * ticksPerFastStep;

if cnt_raw >= HalfPwmPeriod
    cnt_next = HalfPwmPeriod - (cnt_raw - HalfPwmPeriod);
    dir_next = -1;
elseif cnt_raw <= 0
    cnt_next = -cnt_raw;
    dir_next = 1;
else
    cnt_next = cnt_raw;
    dir_next = dir_prev;
end

end

== matlab function FOC_ctrl/PWM_PhaseCurrent/PWM_Carrier/2x dead time ==
  data: cnt input; gate_H output; dir input; ccrUp input; ccrDown input; hiRaw_prev input double; stepsSinceEdge_prev input double; deadTimeFastSteps input; gate_L output; hiRaw_next output; stepsSinceEdge_next output
function [gate_H, gate_L, hiRaw_next, stepsSinceEdge_next] = ss_pwm_gate_step( ...
    cnt, dir, ccrUp, ccrDown, hiRaw_prev, stepsSinceEdge_prev, deadTimeFastSteps)
%SS_PWM_GATE_STEP One fast-rate (p.FastTs) step of a single phase's
% high/low-side switch state, matching STM32 timer PWM mode 1 (active
% while counter < compare value, regardless of counting direction) with
% dead-time inserted around every transition.
%
% Call this once per phase (A/B/C) each fast step - each phase has its
% own hiRaw_prev/stepsSinceEdge_prev state, fed back through Unit Delay
% (Z^-1) blocks AT THE FAST RATE, initial condition hiRaw=false,
% stepsSinceEdge=deadTimeFastSteps (so the very first step isn't wrongly
% held in a dead zone).
%
% This is a genuinely stateful, one-fast-step-at-a-time replacement for
% ss_pwm_waveform.m's batch/offline NxN dead-time trick - simpler and
% more natural now that this runs as part of the live simulation instead
% of a one-shot reconstruction: "how many fast steps since the last
% transition" is just a counter, no need to find edges after the fact.
%
% cnt, dir            : ss_pwm_carrier_step.m output, this fast step
% ccrUp, ccrDown       : this phase's compare value for the up-count/
%                        down-count half (ss_calc_duty_and_samplepoints.m's
%                        DmaBuffCCR_up(k)/DmaBuffCCR_down(k), HELD constant
%                        across the whole PWM period via a Rate Transition
%                        block from the slow p.Ts domain)
% hiRaw_prev           : previous fast step's un-gated compare result
%                        (before dead-time), for edge detection
% stepsSinceEdge_prev  : fast steps elapsed since the last transition
% deadTimeFastSteps    : p.DeadTimeFastSteps
%
% gate_H, gate_L       : dead-time-gated high/low-side switch state
% hiRaw_next, stepsSinceEdge_next : feed back to next fast step

if dir > 0
    hiRaw_next = double(cnt < ccrUp);
else
    hiRaw_next = double(cnt < ccrDown);
end

if hiRaw_next ~= hiRaw_prev
    stepsSinceEdge_next = double(0);
else
    stepsSinceEdge_next = double(stepsSinceEdge_prev + 1);
end

inDeadZone = stepsSinceEdge_next <= deadTimeFastSteps;

gate_H = double(hiRaw_next & ~inDeadZone);
gate_L = double(~hiRaw_next & ~inDeadZone);

end

== matlab function FOC_ctrl/PWM_PhaseCurrent/PWM_Carrier/MATLAB Function2 ==
  data: cnt input; gate_H output double; dir input; ccrUp input; ccrDown input; hiRaw_prev input double; stepsSinceEdge_prev input double; deadTimeFastSteps input; gate_L output double; hiRaw_next output; stepsSinceEdge_next output
function [gate_H, gate_L, hiRaw_next, stepsSinceEdge_next] = ss_pwm_gate_step( ...
    cnt, dir, ccrUp, ccrDown, hiRaw_prev, stepsSinceEdge_prev, deadTimeFastSteps)
%SS_PWM_GATE_STEP One fast-rate (p.FastTs) step of a single phase's
% high/low-side switch state, matching STM32 timer PWM mode 1 (active
% while counter < compare value, regardless of counting direction) with
% dead-time inserted around every transition.
%
% Call this once per phase (A/B/C) each fast step - each phase has its
% own hiRaw_prev/stepsSinceEdge_prev state, fed back through Unit Delay
% (Z^-1) blocks AT THE FAST RATE, initial condition hiRaw=false,
% stepsSinceEdge=deadTimeFastSteps (so the very first step isn't wrongly
% held in a dead zone).
%
% This is a genuinely stateful, one-fast-step-at-a-time replacement for
% ss_pwm_waveform.m's batch/offline NxN dead-time trick - simpler and
% more natural now that this runs as part of the live simulation instead
% of a one-shot reconstruction: "how many fast steps since the last
% transition" is just a counter, no need to find edges after the fact.
%
% cnt, dir            : ss_pwm_carrier_step.m output, this fast step
% ccrUp, ccrDown       : this phase's compare value for the up-count/
%                        down-count half (ss_calc_duty_and_samplepoints.m's
%                        DmaBuffCCR_up(k)/DmaBuffCCR_down(k), HELD constant
%                        across the whole PWM period via a Rate Transition
%                        block from the slow p.Ts domain)
% hiRaw_prev           : previous fast step's un-gated compare result
%                        (before dead-time), for edge detection
% stepsSinceEdge_prev  : fast steps elapsed since the last transition
% deadTimeFastSteps    : p.DeadTimeFastSteps
%
% gate_H, gate_L       : dead-time-gated high/low-side switch state
% hiRaw_next, stepsSinceEdge_next : feed back to next fast step

if dir > 0
    hiRaw_next = double(cnt < ccrUp);
else
    hiRaw_next = double(cnt < ccrDown);
end

if hiRaw_next ~= hiRaw_prev
    stepsSinceEdge_next = double(0);
else
    stepsSinceEdge_next = double(stepsSinceEdge_prev + 1);
end

inDeadZone = stepsSinceEdge_next < deadTimeFastSteps;

gate_H = double(hiRaw_next & ~inDeadZone);
gate_L = double(~hiRaw_next & ~inDeadZone);

end

== matlab function FOC_ctrl/PWM_PhaseCurrent/PWM_Carrier/MATLAB Function3 ==
  data: cnt input; gate_H output double; dir input; ccrUp input; ccrDown input; hiRaw_prev input double; stepsSinceEdge_prev input double; deadTimeFastSteps input; gate_L output double; hiRaw_next output; stepsSinceEdge_next output
function [gate_H, gate_L, hiRaw_next, stepsSinceEdge_next] = ss_pwm_gate_step( ...
    cnt, dir, ccrUp, ccrDown, hiRaw_prev, stepsSinceEdge_prev, deadTimeFastSteps)
%SS_PWM_GATE_STEP One fast-rate (p.FastTs) step of a single phase's
% high/low-side switch state, matching STM32 timer PWM mode 1 (active
% while counter < compare value, regardless of counting direction) with
% dead-time inserted around every transition.
%
% Call this once per phase (A/B/C) each fast step - each phase has its
% own hiRaw_prev/stepsSinceEdge_prev state, fed back through Unit Delay
% (Z^-1) blocks AT THE FAST RATE, initial condition hiRaw=false,
% stepsSinceEdge=deadTimeFastSteps (so the very first step isn't wrongly
% held in a dead zone).
%
% This is a genuinely stateful, one-fast-step-at-a-time replacement for
% ss_pwm_waveform.m's batch/offline NxN dead-time trick - simpler and
% more natural now that this runs as part of the live simulation instead
% of a one-shot reconstruction: "how many fast steps since the last
% transition" is just a counter, no need to find edges after the fact.
%
% cnt, dir            : ss_pwm_carrier_step.m output, this fast step
% ccrUp, ccrDown       : this phase's compare value for the up-count/
%                        down-count half (ss_calc_duty_and_samplepoints.m's
%                        DmaBuffCCR_up(k)/DmaBuffCCR_down(k), HELD constant
%                        across the whole PWM period via a Rate Transition
%                        block from the slow p.Ts domain)
% hiRaw_prev           : previous fast step's un-gated compare result
%                        (before dead-time), for edge detection
% stepsSinceEdge_prev  : fast steps elapsed since the last transition
% deadTimeFastSteps    : p.DeadTimeFastSteps
%
% gate_H, gate_L       : dead-time-gated high/low-side switch state
% hiRaw_next, stepsSinceEdge_next : feed back to next fast step

if dir > 0
    hiRaw_next = double(cnt < ccrUp);
else
    hiRaw_next = double(cnt < ccrDown);
end

if hiRaw_next ~= hiRaw_prev
    stepsSinceEdge_next = double(0);
else
    stepsSinceEdge_next = double(stepsSinceEdge_prev + 1);
end

inDeadZone = stepsSinceEdge_next < deadTimeFastSteps;

gate_H = double(hiRaw_next & ~inDeadZone);
gate_L = double(~hiRaw_next & ~inDeadZone);

end

== matlab function FOC_ctrl/PWM_PhaseCurrent/PWM_Carrier/MATLAB Function4 ==
  data: cnt input; gate_H output double; dir input; ccrUp input; ccrDown input; hiRaw_prev input double; stepsSinceEdge_prev input double; deadTimeFastSteps input; gate_L output double; hiRaw_next output; stepsSinceEdge_next output
function [gate_H, gate_L, hiRaw_next, stepsSinceEdge_next] = ss_pwm_gate_step( ...
    cnt, dir, ccrUp, ccrDown, hiRaw_prev, stepsSinceEdge_prev, deadTimeFastSteps)
%SS_PWM_GATE_STEP One fast-rate (p.FastTs) step of a single phase's
% high/low-side switch state, matching STM32 timer PWM mode 1 (active
% while counter < compare value, regardless of counting direction) with
% dead-time inserted around every transition.
%
% Call this once per phase (A/B/C) each fast step - each phase has its
% own hiRaw_prev/stepsSinceEdge_prev state, fed back through Unit Delay
% (Z^-1) blocks AT THE FAST RATE, initial condition hiRaw=false,
% stepsSinceEdge=deadTimeFastSteps (so the very first step isn't wrongly
% held in a dead zone).
%
% This is a genuinely stateful, one-fast-step-at-a-time replacement for
% ss_pwm_waveform.m's batch/offline NxN dead-time trick - simpler and
% more natural now that this runs as part of the live simulation instead
% of a one-shot reconstruction: "how many fast steps since the last
% transition" is just a counter, no need to find edges after the fact.
%
% cnt, dir            : ss_pwm_carrier_step.m output, this fast step
% ccrUp, ccrDown       : this phase's compare value for the up-count/
%                        down-count half (ss_calc_duty_and_samplepoints.m's
%                        DmaBuffCCR_up(k)/DmaBuffCCR_down(k), HELD constant
%                        across the whole PWM period via a Rate Transition
%                        block from the slow p.Ts domain)
% hiRaw_prev           : previous fast step's un-gated compare result
%                        (before dead-time), for edge detection
% stepsSinceEdge_prev  : fast steps elapsed since the last transition
% deadTimeFastSteps    : p.DeadTimeFastSteps
%
% gate_H, gate_L       : dead-time-gated high/low-side switch state
% hiRaw_next, stepsSinceEdge_next : feed back to next fast step

if dir > 0
    hiRaw_next = double(cnt < ccrUp);
else
    hiRaw_next = double(cnt < ccrDown);
end

if hiRaw_next ~= hiRaw_prev
    stepsSinceEdge_next = double(0);
else
    stepsSinceEdge_next = double(stepsSinceEdge_prev + 1);
end

inDeadZone = stepsSinceEdge_next < deadTimeFastSteps;

gate_H = double(hiRaw_next & ~inDeadZone);
gate_L = double(~hiRaw_next & ~inDeadZone);

end
